simulink model "exemploZoH"  (R2024b)
settings: Solver=VariableStepAuto  StartTime=0.0  StopTime=0.02  RelTol=1e-3
libraries: spsSampleandHoldLib x1
settings Model: Creator=Juan  LastModifiedBy=darla
settings SolverCC: AlgebraicLoopSolver=TrustRegion
settings DataIOCC: ReturnWorkspaceOutputs=off
settings DebuggingCC: UnconnectedInputMsg=warning  UnconnectedOutputMsg=warning  UnconnectedLineMsg=warning  ArithmeticOperatorsInVariantConditions=warning
settings ModelReferenceCC: EnableRefExpFcnMdlSchedulingChecks=on
settings SFSimCC: SimUseLocalCustomCode=off  CustomCodeUndefinedFunction=UseInterfaceOnly
settings RTWCC: RTWUseLocalCustomCode=off  GPUComputeCapability=3.5

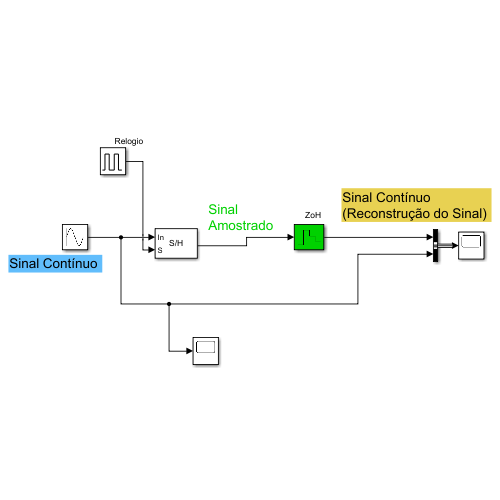
[thumbnail: Simulink's stored preview of the top-level diagram]
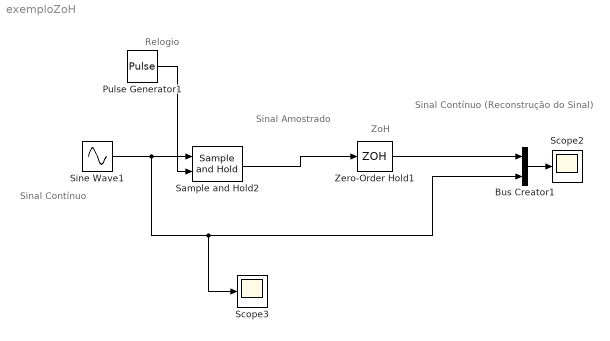
== system exemploZoH ==
  note: Sinal Contínuo
  note: Relogio
  note: ZoH
  note: Sinal Contínuo
      | (Reconstrução do Sinal)
  note: Sinal
      | Amostrado
  Bus Creator1 : BusCreator  Inputs=2
  Pulse Generator1 : DiscretePulseGenerator  PulseType=Time based  Period=1e-3  PulseWidth=50
  Sample and Hold2 : spsSampleandHoldLib/Sample and Hold  ic=0  Ts=1e-3
      settings: LibrarySourceBlock=|
      | sps_lib/Control/Sample and
      | Hold
  Scope2 : Scope
  Scope3 : Scope
  Sine Wave1 : Sin  Frequency=2*pi*100  SampleTime=0
  Zero-Order Hold1 : ZeroOrderHold  SampleTime=1e-3
  wires:
  Bus Creator1/1 -> Scope2/1
  Zero-Order Hold1/1 -> Bus Creator1/1
  Sine Wave1/1 -> Sample and Hold2/1, Scope3/1, Bus Creator1/2
  Pulse Generator1/1 -> Sample and Hold2/2
  Sample and Hold2/1 -> Zero-Order Hold1/1
